simulink model "PID_spring_mass_damper_model"  (R2018b)
settings: Solver=ode45  StartTime=0.0  StopTime=60  MaxStep=deltaTMax  RelTol=1e-3  EnableMultiTasking=on
values from neighbouring files (symbols this model uses):
  A = [0 1;-k/m -c/m]    [MAIN_PID_spring_mass_damper.m]
  B = [0;1/m]    [MAIN_PID_spring_mass_damper.m]
  C = [1 0]    [MAIN_PID_spring_mass_damper.m]
  D = [0]    [MAIN_PID_spring_mass_damper.m]
  KD = 0.6    [MAIN_PID_spring_mass_damper.m]
  KI = 0.15    [MAIN_PID_spring_mass_damper.m]
  KP = 1.2    [MAIN_PID_spring_mass_damper.m]
  p = 0.01    [MAIN_PID_spring_mass_damper.m]
  x0 = [0;0]    [MAIN_PID_spring_mass_damper.m]
  xILimit = 1000    [MAIN_PID_spring_mass_damper.m]
settings Model: Creator=lum  LastModifiedBy=Christopher
settings DataIOCC: LimitDataPoints=on  SaveFormat=Array  SignalLoggingSaveFormat=ModelDataLogs
settings OptimizationCC: ExpressionDepthLimit=2147483647  LifeSpan=inf
settings DebuggingCC: UnderspecifiedInitializationDetection=Classic  MergeDetectMultiDrivingBlocksExec=none  SolverPrmCheckMsg=warning  FcnCallInpInsideContextMsg=warning  StateNameClashWarn=warning  SFUnexpectedBacktrackingDiag=warning  SFNoUnconditionalDefaultTransitionDiag=warning  SFExecutionAtInitializationDiag=none
settings HardwareCC: ProdBitPerPointer=32  ProdBitPerSizeT=32  ProdBitPerPtrDiffT=32  ProdLargestAtomicFloat=None  ProdIntDivRoundTo=Undefined  ProdEndianess=Unspecified  ProdWordSize=32  ProdHWDeviceType=32-bit Generic
settings ModelReferenceCC: PropagateSignalLabelsOutOfModel=off
settings SFSimCC: SimUseLocalCustomCode=off
settings RTWCC: RTWUseLocalCustomCode=off
settings CodeAppCC: StateflowObjectComments=on
settings GRTTargetCC: TargetLangStandard=C89/C90 (ANSI)  GeneratePreprocessorConditionals=Disable all  CombineOutputUpdateFcns=off  GRTInterface=on
settings ConfigComp: CovMetricSettings=dw  CovHtmlReporting=on  CovSaveCumulativeToWorkspaceVar=on  CovSaveSingleToWorkspaceVar=on  CovExternalEMLEnable=off

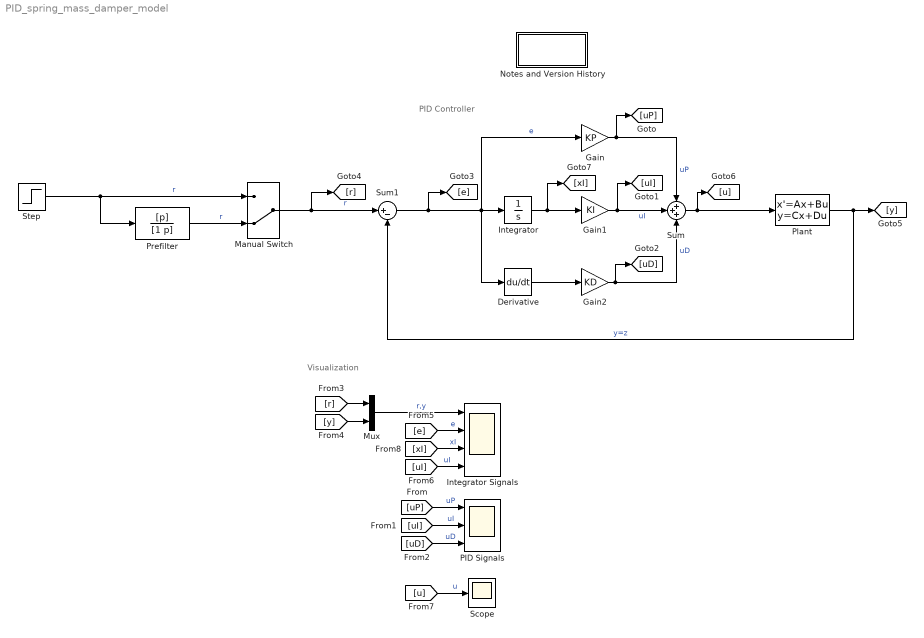
== system PID_spring_mass_damper_model ==
  note: Visualization
  note: PID Controller
  Derivative : Derivative
  Gain : Gain  Gain=KP
  Gain1 : Gain  Gain=KI
  Gain2 : Gain  Gain=KD
  Integrator : Integrator  LimitOutput=on  UpperSaturationLimit=xILimit  LowerSaturationLimit=-xILimit
  Integrator Signals : Scope  NumInputPorts=4
  Manual Switch : ManualSwitch  CurrentSetting=0
  Mux : Mux  Inputs=2
  Notes and Version History : Subsystem
  PID Signals : Scope  NumInputPorts=3
  Plant : StateSpace  A=A  B=B  C=C  D=D  InitialCondition=x0
  Prefilter : TransferFcn  Numerator=[p]  Denominator=[1 p]
  Scope : Scope
  Step : Step  SampleTime=0
  Sum : Sum  Inputs=+++
  Sum1 : Sum  Inputs=|+-
  wires:
  Plant/1 -> Sum1/2, [y]  "y=z"
  Gain/1 -> Sum/1, [uP]  "uP"
  Manual Switch/1 -> [r], Sum1/1  "r"
  Sum1/1 -> [e], Derivative/1, Gain/1, Integrator/1  "e"
  Sum/1 -> [u], Plant/1
  Integrator/1 -> [xI], Gain1/1
  Gain1/1 -> [uI], Sum/2  "uI"
  Derivative/1 -> Gain2/1
  Gain2/1 -> [uD], Sum/3  "uD"
  [uP] -> PID Signals/1  "uP"
  [uI] -> PID Signals/2  "uI"
  [uD] -> PID Signals/3  "uD"
  Mux/1 -> Integrator Signals/1  "r,y"
  [r] -> Mux/1
  [y] -> Mux/2
  [e] -> Integrator Signals/2  "e"
  [uI] -> Integrator Signals/4  "uI"
  [u] -> Scope/1  "u"
  Step/1 -> Prefilter/1, Manual Switch/1  "r"
  Prefilter/1 -> Manual Switch/2  "r"
  [xI] -> Integrator Signals/3  "xI"

== system PID_spring_mass_damper_model/Notes and Version History ==
  note: Illustrate PID control
      |
      | Christopher Lum
      | lum@uw.edu
      |
      | Version History
      | 05/112/21: Created
